simulink model "controllers"  (Simulink 6.3)
settings: Solver=ode45  StartTime=0.0  StopTime=10.0  RelTol=1e-3
values from neighbouring files (symbols this model uses):
  b = 100    [parameters.m]
  dT = 0.01    [parameters.m]
  m = 2000    [parameters.m]
  V_Ki = 50    [parameters.m]
  V_Kp = 5000    [parameters.m]
settings Model: LastModifiedBy=ericjw

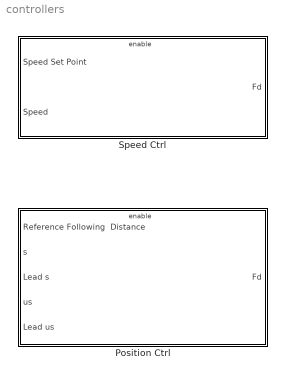
== system controllers ==
  Position Ctrl : Subsystem  TreatAsAtomicUnit=on
  Speed Ctrl : Subsystem  TreatAsAtomicUnit=on

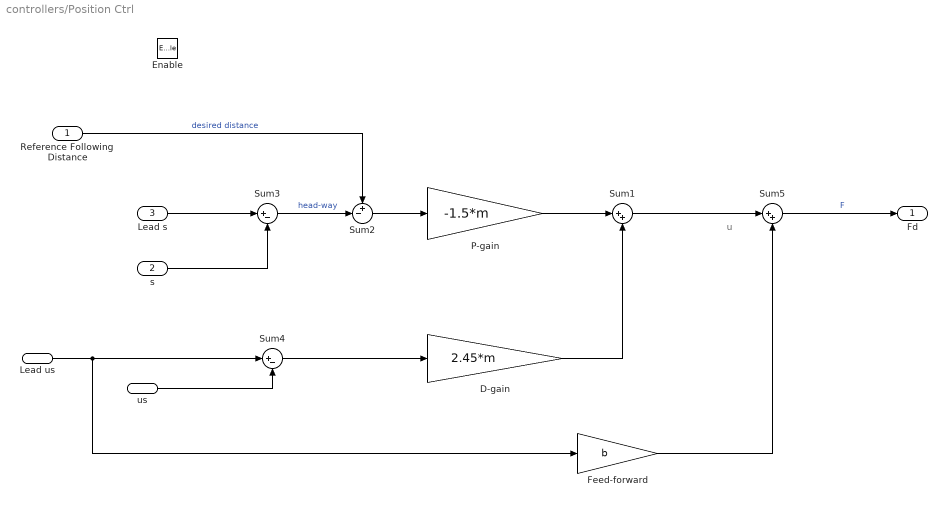
== system controllers/Position Ctrl ==
  note: u
  Reference Following  Distance : Inport
  s : Inport  Port=2
  Lead s : Inport  Port=3
  us : Inport  Port=4
  Lead us : Inport  Port=5
  Enable : EnablePort
  D-gain : Gain  Gain=2.45*m  SaturateOnIntegerOverflow=on
  Feed-forward : Gain  Gain=b  SaturateOnIntegerOverflow=on
  P-gain : Gain  Gain=-1.5*m  SaturateOnIntegerOverflow=on
  Sum1 : Sum  Inputs=|++  SaturateOnIntegerOverflow=on
  Sum2 : Sum  Inputs=+-|  SaturateOnIntegerOverflow=on
  Sum3 : Sum  Inputs=|+-  SaturateOnIntegerOverflow=on
  Sum4 : Sum  Inputs=|+-  SaturateOnIntegerOverflow=on
  Sum5 : Sum  Inputs=|++  SaturateOnIntegerOverflow=on
  Fd : Outport
  wires:
  Lead s/1 -> Sum3/1
  s/1 -> Sum3/2
  Reference Following  Distance/1 -> Sum2/1  "desired distance"
  Sum3/1 -> Sum2/2  "head-way"
  Sum2/1 -> P-gain/1
  P-gain/1 -> Sum1/1
  D-gain/1 -> Sum1/2
  us/1 -> Sum4/2
  Lead us/1 -> Sum4/1, Feed-forward/1
  Sum4/1 -> D-gain/1
  Feed-forward/1 -> Sum5/2
  Sum5/1 -> Fd/1  "F"
  Sum1/1 -> Sum5/1

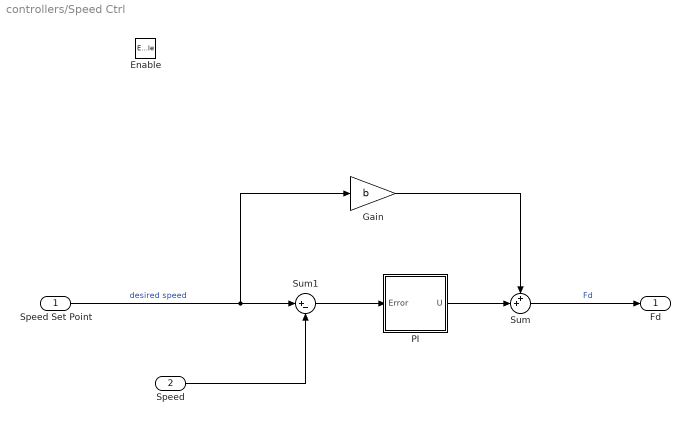
== system controllers/Speed Ctrl ==
  Speed Set Point : Inport
  Speed : Inport  Port=2
  Enable : EnablePort
  Gain : Gain  Gain=b  SaturateOnIntegerOverflow=on
  PI : Subsystem
  Sum : Sum  Inputs=++|  SaturateOnIntegerOverflow=on
  Sum1 : Sum  Inputs=|+-  SaturateOnIntegerOverflow=on
  Fd : Outport
  wires:
  Sum/1 -> Fd/1  "Fd"
  Speed Set Point/1 -> Gain/1, Sum1/1  "desired speed"
  Speed/1 -> Sum1/2
  Sum1/1 -> PI/1(Error)
  Gain/1 -> Sum/1
  PI/1(U) -> Sum/2

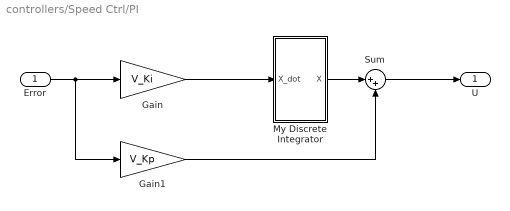
== system controllers/Speed Ctrl/PI ==
  Error : Inport
  Gain : Gain  Gain=V_Ki  SaturateOnIntegerOverflow=on
  Gain1 : Gain  Gain=V_Kp  SaturateOnIntegerOverflow=on
  My Discrete Integrator : Subsystem
  Sum : Sum  Inputs=|++  SaturateOnIntegerOverflow=on
  U : Outport
  wires:
  Gain/1 -> My Discrete Integrator/1(X_dot)
  My Discrete Integrator/1(X) -> Sum/1
  Gain1/1 -> Sum/2
  Error/1 -> Gain/1, Gain1/1
  Sum/1 -> U/1

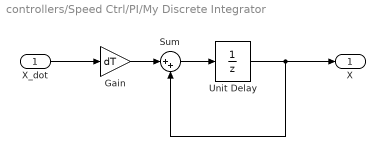
== system controllers/Speed Ctrl/PI/My Discrete Integrator ==
  X_dot : Inport
  Gain : Gain  Gain=dT  SaturateOnIntegerOverflow=on
  Sum : Sum  Inputs=|++  SaturateOnIntegerOverflow=on  InputSameDT=on
  Unit Delay : UnitDelay  SampleTime=-1
  X : Outport
  wires:
  Unit Delay/1 -> X/1, Sum/2
  Sum/1 -> Unit Delay/1
  X_dot/1 -> Gain/1
  Gain/1 -> Sum/1
